simulink model "TestController"  (R2022b)
settings: Solver=FixedStepAuto  StartTime=0.0  StopTime=10.0  RelTol=1e-3
settings Model: Creator=hollis  LastModifiedBy=hunter
settings OptimizationCC: DefaultParameterBehavior=Inlined  EnhancedBackFolding=on  PassReuseOutputArgsAs=Individual arguments  ZeroExternalMemoryAtStartup=off  ZeroInternalMemoryAtStartup=off  OptimizeBlockOrder=speed  DifferentSizesBufferReuse=on  OptimizationCustomize=off  EfficientTunableParamExpr=on
settings DebuggingCC: ParameterTunabilityLossMsg=error
settings HardwareCC: TargetBitPerLong=64  TargetBitPerPointer=64  TargetBitPerSizeT=64  TargetBitPerPtrDiffT=64  TargetLongLongMode=on  TargetIntDivRoundTo=Zero  TargetEndianess=LittleEndian  TargetWordSize=64  TargetHWDeviceType=MATLAB Host  ProdEqTarget=off
settings SFSimCC: MATLABDynamicMemAlloc=off
settings RTWCC: Description=Embedded Coder (host-based shared library target)  SystemTargetFile=ert_shrlib.tlc  GenCodeOnly=on  TemplateMakefile=ert_default_tmf  Toolchain=GNU gcc/g++ | CMake/gmake (64-bit Linux)  BuildConfiguration=Specify
settings CodeAppCC: ForceParamTrailComments=on  IgnoreCustomStorageClasses=off  OperatorAnnotations=on  SimulinkDataObjDesc=on  SFDataObjDesc=on  InsertBlockDesc=on
settings STFCustomTargetCC: TargetLangStandard=C99 (ISO)  MultiwordLength=256  GenerateSampleERTMain=on  ParMdlRefBuildCompliant=on  CompOptLevelCompliant=on  CombineOutputUpdateFcns=on  ERTCustomFileBanners=on  SupportNonInlinedSFcns=off  RemoveResetFunc=on  MATLABClassNameForMDSCustomization=Simulink.SoftwareTarget.ERTCustomization  ModelStepFunctionPrototypeControlCompliant=on  UseToolchainInfoCompliant=on  SystemTargetFile=ert_shrlib.tlc
settings ERTTargetCC: TargetLangStandard=C99 (ISO)  GenerateSampleERTMain=on  ConcurrentExecutionCompliant=off  SupportContinuousTime=on  CPPClassGenCompliant=off  InlinedParameterPlacement=NonHierarchical  ERTCustomFileTemplate=example_file_process.tlc

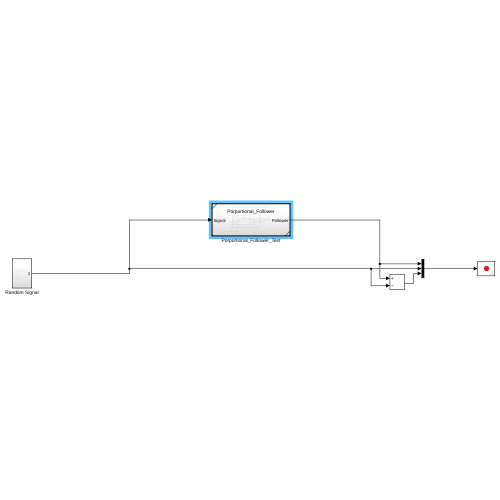
[thumbnail: Simulink's stored preview of the top-level diagram]
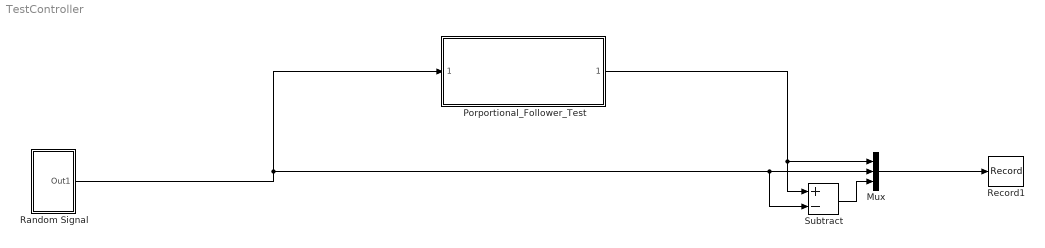
== system TestController ==
  Mux : Mux  Inputs=3
  Porportional_Follower_Test : Subsystem  TreatAsAtomicUnit=on  ReferencedSubsystem=Porportional_Follower
  Random Signal : Subsystem
  Record1 : Record  FileSettingsInternal="{\"entries\":[{\"content\":{\"excelSettings\":{\"content\":{},\"type\":\"Streamout.ExcelSettings\"}},\"type\":\"Streamout.FileSettingStorage\",\"uuid\":\"667a1efb-0bed-49e8-a980-4118dc37b532\"}],\"packageUris\":[\"http://schema.mathworks.com/mf0/streamout_blocks/R2020a\"],\"version\":\"1.0\"}"  Layout=[1 1]  SignalsInternal="{\"entries\":[{\"content\":{\"signals\":[{\"content\":{\"blockPath\":[\"TestController/Record1\"],\"channel\":[],\"dimensions\":[3],\"domain\":\"TestController/Record1\",\"hasChildren\":true,\"lineColor\":\"#d95319\",\"plots\":[],\"port\":1,\"sid\":[],\"signalID\":8,\"signalName\":\"Mux\"},\"type\":\"RecordBlkView.Signal\",\"uuid\":\"6a8494f1-7408-4556-a11c-dd35229971ca\"},{\"content\":{\"blockPath\":[\"TestController/Record1\"],\"channel\":[1],\"dimensions\":[3],\"domain\":\"TestController/Record1\",\"lineColor\":\"#fe330a\",\"parentID\":8,\"plots\":[1],\"port\":1,\"sid\":[],\"signalID\":9,\"signalName\":\"Mux\"},\"type\":\"RecordBlkView.Signal\",\"uuid\":\"1409f04b-d067-4dbf-b92d-cf8560dd0879\"},{\"content\":{\"blockPath\":[\"TestController/Record1\"],\"channel\":[2],\"dimensions\":[3],\"domain\":\"TestController/Record1\",\"lineColor\":\"#22b573\",\"parentID\":8,\"plots\":[1],\"port\":1,\"sid\":[],\"signalID\":10,\"signalName\":\"Mux\"},\"type\":\"RecordBlkView.Signal\",\"uuid\":\"27bd8faa-e88c-4fb5-b393-39009d643369\"},{\"content\":{\"blockPath\":[\"TestController/Record1\"],\"channel\":[3],\"dimensions\":[3],\"domain\":\"TestController/Record1\",\"lineColor\":\"#b746ff\",\"parentID\":8,\"plots\":[1],\"port\":1,\"sid\":[],\"signalID\":11,\"signalName\":\"Mux\"},\"type\":\"RecordBlkView.Signal\",\"uuid\":\"520f8d2a-8da9-4771-ad23-24cda621cbe9\"}]},\"type\":\"RecordBlkView.InputSignals\",\"uuid\":\"d9504e5e-970e-4d13-b1c4-1f014de30b92\"}],\"packageUris\":[\"http://schema.mathworks.com/mf0/streamout_blocks/R2020a\"],\"version\":\"1.0\"}"  VisualizationBindings="{\"sparklinesplugin\":{\"info\":[{\"bindingParametersList\":[],\"subplotID\":1}]}}"
  Subtract : Sum  Inputs=+-
  wires:
  Random Signal/1(Out1) -> Porportional_Follower_Test/1, Subtract/2, Mux/2
  Mux/1 -> Record1/1
  Porportional_Follower_Test/1 -> Subtract/1, Mux/1
  Subtract/1 -> Mux/3

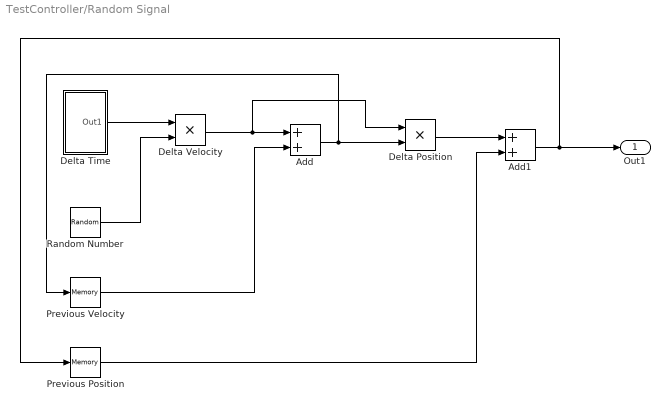
== system TestController/Random Signal ==
  Add : Sum
  Add1 : Sum
  Delta Position : Product
  Delta Time : Subsystem
  Delta Velocity : Product
  Previous Position : Memory
  Previous Velocity : Memory
  Random Number : RandomNumber  Variance=10  Seed=8  SampleTime=0.1
  Out1 : Outport
  wires:
  Previous Position/1 -> Add1/2
  Random Number/1 -> Delta Velocity/2
  Add/1 -> Delta Position/2, Previous Velocity/1
  Delta Position/1 -> Add1/1
  Previous Velocity/1 -> Add/2
  Delta Velocity/1 -> Delta Position/1, Add/1
  Delta Time/1(Out1) -> Delta Velocity/1
  Add1/1 -> Out1/1, Previous Position/1

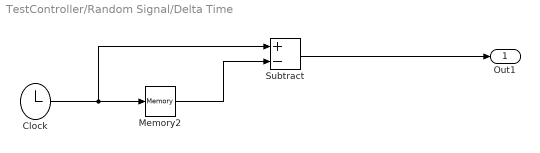
== system TestController/Random Signal/Delta Time ==
  Clock : Clock
  Memory2 : Memory
  Subtract : Sum  Inputs=+-
  Out1 : Outport
  wires:
  Memory2/1 -> Subtract/2
  Clock/1 -> Subtract/1, Memory2/1
  Subtract/1 -> Out1/1
